simulink model "FIR_filter_shell"  (R2020b)
settings: Solver=FixedStepDiscrete  StartTime=0.0  StopTime=10.0  RelTol=1e-3
model workspace: external: MATLAB File /home/mcrisafu/ddm/mcrisafu_test01/matlab/lib_FIR_filter/models/FIR_variables.m (data not in the file)
values from neighbouring files (symbols this model uses):
  b = fir1(n,[Wlow Whigh],'DC-0')    [FIR_variables.m]
settings Model: DataTypeOverride=Off  VariantFading=off  OrderedModelArguments=off  Creator=mcrisafu  LastModifiedBy=mcrisafu
settings OptimizationCC: BlockReduction=off  ConditionallyExecuteInputs=off  DefaultParameterBehavior=Inlined
settings DebuggingCC: AlgebraicLoopMsg=error  SingleTaskRateTransMsg=error
settings HardwareCC: ProdBitPerPointer=32  ProdBitPerSizeT=32  ProdBitPerPtrDiffT=32  ProdLargestAtomicFloat=None  ProdIntDivRoundTo=Undefined  ProdEndianess=Unspecified  ProdWordSize=32  ProdHWDeviceType=ASIC/FPGA->ASIC/FPGA  TargetBitPerLong=64  TargetBitPerPointer=64  TargetBitPerSizeT=64  TargetBitPerPtrDiffT=64  TargetLongLongMode=on  TargetIntDivRoundTo=Zero  TargetEndianess=LittleEndian  TargetWordSize=64  TargetHWDeviceType=Custom Processor->MATLAB Host Computer  ProdEqTarget=off

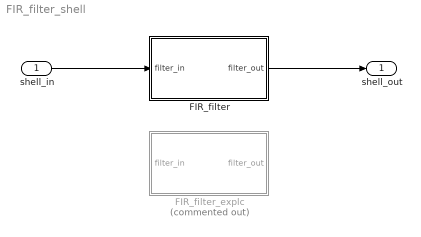
== system FIR_filter_shell ==
  shell_in : Inport  OutMin=[-1]  OutMax=[1]  OutDataTypeStr=fixdt(1,24)
  FIR_filter : Subsystem
  FIR_filter_explc : Subsystem  Commented=on
  shell_out : Outport
  wires:
  shell_in/1 -> FIR_filter/1(filter_in)
  FIR_filter/1(filter_out) -> shell_out/1

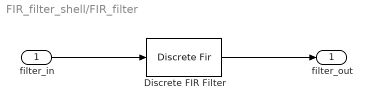
== system FIR_filter_shell/FIR_filter ==
  filter_in : Inport
  Discrete FIR Filter : DiscreteFir  Coefficients=b  OutMin=[-1]  OutMax=[1]  OutDataTypeStr=fixdt(1,24)
  filter_out : Outport  OutMin=[-1]  OutMax=[1]  OutDataTypeStr=fixdt(1,24)
  wires:
  filter_in/1 -> Discrete FIR Filter/1
  Discrete FIR Filter/1 -> filter_out/1

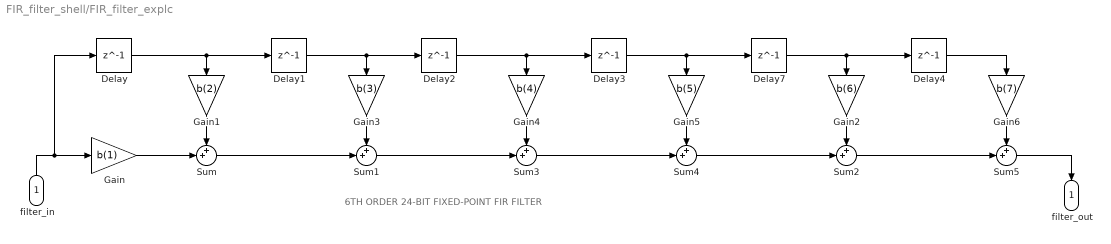
== system FIR_filter_shell/FIR_filter_explc ==
  note: 6TH ORDER 24-BIT FIXED-POINT FIR FILTER
  filter_in : Inport
  Delay{,1..4,7} (6 alike) : Delay  DelayLength=1
  Gain : Gain  Gain=b(1)  OutMin=[-1]  OutMax=[1]  OutDataTypeStr=fixdt(1,24)
  Gain1 : Gain  Gain=b(2)  OutMin=[-1]  OutMax=[1]  OutDataTypeStr=fixdt(1,24)
  Gain2 : Gain  Gain=b(6)  OutMin=[-1]  OutMax=[1]  OutDataTypeStr=fixdt(1,24)
  Gain3 : Gain  Gain=b(3)  OutMin=[-1]  OutMax=[1]  OutDataTypeStr=fixdt(1,24)
  Gain4 : Gain  Gain=b(4)  OutMin=[-1]  OutMax=[1]  OutDataTypeStr=fixdt(1,24)
  Gain5 : Gain  Gain=b(5)  OutMin=[-1]  OutMax=[1]  OutDataTypeStr=fixdt(1,24)
  Gain6 : Gain  Gain=b(7)  OutMin=[-1]  OutMax=[1]  OutDataTypeStr=fixdt(1,24)
  Sum{,1..5} (6 alike) : Sum  Inputs=++|  OutMin=[-1]  OutMax=[1]  OutDataTypeStr=Inherit: Inherit via back propagation
  filter_out : Outport  OutMin=[-1]  OutMax=[1]  OutDataTypeStr=fixdt(1,24)
  wires:
  Gain/1 -> Sum/2
  filter_in/1 -> Gain/1, Delay/1
  Delay/1 -> Gain1/1, Delay1/1
  Gain3/1 -> Sum1/1
  Delay1/1 -> Delay2/1, Gain3/1
  Sum/1 -> Sum1/2
  Gain1/1 -> Sum/1
  Sum3/1 -> Sum4/2
  Gain5/1 -> Sum4/1
  Delay3/1 -> Delay7/1, Gain5/1
  Delay2/1 -> Gain4/1, Delay3/1
  Sum1/1 -> Sum3/2
  Gain4/1 -> Sum3/1
  Gain2/1 -> Sum2/1
  Sum2/1 -> Sum5/2
  Gain6/1 -> Sum5/1
  Delay4/1 -> Gain6/1
  Sum4/1 -> Sum2/2
  Delay7/1 -> Gain2/1, Delay4/1
  Sum5/1 -> filter_out/1
